simulink model "heat25830_staliro_01"  (Simulink 9.2)
settings: Solver=FixedStepAuto  StartTime=0.0  StopTime=50  FixedStep=0.05  RelTol=1e-5  AbsTol=1e-5  EnableMultiTasking=on
undefined symbols (not defined in the file or in its folder): Amat, bvec, cvec, dif, get, h, rooms, xinit
settings Model: Creator=gfaineko  LastModifiedBy=xxx
settings SolverCC: AutoScaleAbsTol=off
settings DataIOCC: LimitDataPoints=off  SaveOutput=off  SignalLogging=off  DSMLogging=off  SaveTime=off  SignalLoggingName=sigsOut
settings OptimizationCC: ExpressionDepthLimit=2147483647
settings DebuggingCC: SaveWithParameterizedLinksMsg=none  SignalResolutionControl=TryResolveAllWithWarning  MultiTaskDSMMsg=warning  MultiTaskCondExecSysMsg=none  InitInArrayFormatMsg=none
settings HardwareCC: TargetUnknown=on
settings SFSimCC: SimParseCustomCode=off

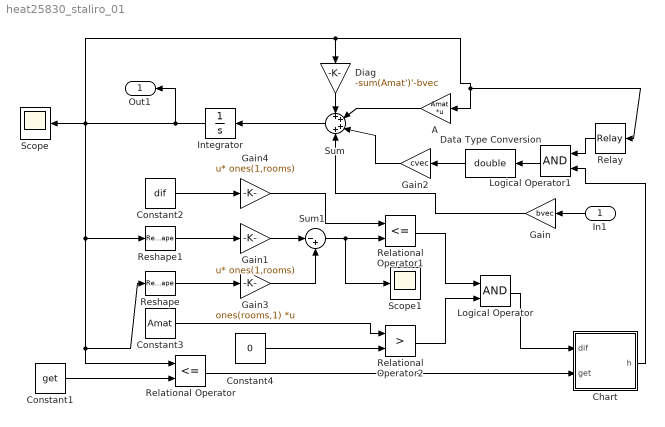
== system heat25830_staliro_01 ==
  In1 : Inport
  A : Gain  Gain=Amat  Multiplication=Matrix(K*u)  SaturateOnIntegerOverflow=on  OutDataTypeStr=Inherit: Same as input  ParamDataTypeStr=Inherit: Same as input
  Chart : Stateflow chart  TreatAsAtomicUnit=on
  Constant1 : Constant  Value=get
  Constant2 : Constant  Value=dif
  Constant3 : Constant  Value=Amat  VectorParams1D=off
  Constant4 : Constant  Value=0
  Data Type Conversion : DataTypeConversion  OutDataTypeStr=double  SaturateOnIntegerOverflow=on  RndMeth=Zero
  Diag : Gain  Gain=-sum(Amat')'-bvec  SaturateOnIntegerOverflow=on  OutDataTypeStr=Inherit: Same as input  ParamDataTypeStr=Inherit: Same as input
  Gain : Gain  Gain=bvec  SaturateOnIntegerOverflow=on  OutDataTypeStr=Inherit: Same as input  ParamDataTypeStr=Inherit: Same as input
  Gain1 : Gain  Gain=ones(1,rooms)  Multiplication=Matrix(u*K)  SaturateOnIntegerOverflow=on  OutDataTypeStr=Inherit: Same as input  ParamDataTypeStr=Inherit: Same as input
  Gain2 : Gain  Gain=cvec  SaturateOnIntegerOverflow=on  OutDataTypeStr=Inherit: Same as input  ParamDataTypeStr=Inherit: Same as input
  Gain3 : Gain  Gain=ones(rooms,1)  Multiplication=Matrix(K*u)  SaturateOnIntegerOverflow=on  OutDataTypeStr=Inherit: Same as input  ParamDataTypeStr=Inherit: Same as input
  Gain4 : Gain  Gain=ones(1,rooms)  Multiplication=Matrix(u*K)  SaturateOnIntegerOverflow=on  OutDataTypeStr=Inherit: Same as input  ParamDataTypeStr=Inherit: Same as input
  Integrator : Integrator  InitialCondition=xinit
  Logical Operator : Logic  AllPortsSameDT=off
  Logical Operator1 : Logic  AllPortsSameDT=off
  Relational Operator : RelationalOperator  Operator=<=  OutDataTypeStr=boolean  RndMeth=Nearest
  Relational Operator1 : RelationalOperator  Operator=<=  OutDataTypeStr=boolean  RndMeth=Nearest
  Relational Operator2 : RelationalOperator  Operator=>  OutDataTypeStr=boolean  RndMeth=Nearest
  Relay : Relay  OnSwitchValue=off  OffSwitchValue=on  OnOutputValue=0  OffOutputValue=1
  Reshape : Reshape  OutputDimensionality=Row vector (2-D)
  Reshape1 : Reshape  OutputDimensionality=Column vector (2-D)
  Scope : Scope
  Scope1 : Scope
  Sum : Sum  Inputs=++++  SaturateOnIntegerOverflow=on
  Sum1 : Sum  Inputs=|-+  SaturateOnIntegerOverflow=on
  Out1 : Outport
  wires:
  Sum/1 -> Integrator/1
  Integrator/1 -> Scope/1, Relational Operator/1, Reshape/1, Reshape1/1, Diag/1, Relay/1, A/1, Out1/1
  Diag/1 -> Sum/1
  Relay/1 -> Logical Operator1/1
  Gain/1 -> Sum/4
  In1/1 -> Gain/1
  Relational Operator/1 -> Chart/2(get)
  Constant1/1 -> Relational Operator/2
  Reshape1/1 -> Gain1/1
  Reshape/1 -> Gain3/1
  Gain1/1 -> Sum1/1
  Gain3/1 -> Sum1/2
  Sum1/1 -> Scope1/1, Relational Operator1/2
  Gain4/1 -> Relational Operator1/1
  Constant2/1 -> Gain4/1
  Relational Operator1/1 -> Logical Operator/1
  Constant3/1 -> Relational Operator2/1
  Constant4/1 -> Relational Operator2/2
  Relational Operator2/1 -> Logical Operator/2
  Logical Operator/1 -> Chart/1(dif)
  Logical Operator1/1 -> Data Type Conversion/1
  Data Type Conversion/1 -> Gain2/1
  Chart/1(h) -> Logical Operator1/2
  A/1 -> Sum/2
  Gain2/1 -> Sum/3

== stateflow chart Chart ==
  state main [parallel]
    settings: executionOrder=1
    (junction 8) -> (junction 6) [order 1] : [id2<rooms]
    (junction 6) -> (junction 10)
    (junction 12) -> (junction 7) [order 1] : [id1<rooms]
    (junction 7) -> (junction 9)
    (junction 9) -> (junction 8) [order 1] : [get[id1]&!h[id1]]
    (junction 10) -> (junction 11) [order 1] : [dif[id1][id2]&h[id2]]
    (junction 13) -> (junction 8)
    (junction 8) -> (junction 15) [order 2] : {id2=0;}
    (junction 9) -> (junction 14) [order 2]
    (junction 10) -> (junction 13) [order 2] : {id2++;}
    (junction 11) -> (junction 18) : {h[id1]=1;h[id2]=0;}
    main -> (junction 12) : {id1=0;id2=0;}
    (junction 16) -> (junction 12)
    (junction 12) -> (junction 17) [order 2]
    (junction 15) -> (junction 14)
    (junction 14) -> (junction 16) : {id1++;}
    (junction 18) -> (junction 17)
    (junction 17) -> main
  data: id1 local int16; id2 local int16; rooms parameter double; dif input boolean size=10,10; get input boolean size=10; h output double size=10 =h
